simulink model "MMAE_leftlaneChange_behavior_identification"  (R2018b)
settings: Solver=FixedStepAuto  StartTime=0.0  StopTime=15  FixedStep=1e-3  RelTol=1e-3
values from neighbouring files (symbols this model uses):
  P_init = 1    [initialization.m]
  Ts_bp = 0.1    [initialization.m]    (also in laneChangeSinusoidalFcn.m = 0.01; laneChangeSinusoidalJacobianFcn.m = 0.01; leftLaneChangeParametricFcn.m = 0.01; leftLaneChangeParametricWithAccFcn.m = 0.01)
  vx = X(2)    [cv_model_fun.m]    (also in initialization.m = 10)
  vy = X(4)    [cv_model_fun.m]    (also in initialization.m = 0)
  x = X(1)    [KinematicBicycleModel.m]    (also in SimplifiedKinematicBicycleModel.m; behavior_model.m = 0:0.01:20; cca_model_fun.m; ctra_model_fun.m)
  y = X(2)    [KinematicBicycleModel.m]    (also in SimplifiedKinematicBicycleModel.m; behavior_model.m = [distances velocities]; cca_model_fun.m; ctra_model_fun.m)
libraries: simulink x5
settings Model: Creator=jasprit  LastModifiedBy=jasprit
settings SFSimCC: SimUseLocalCustomCode=off
settings RTWCC: RTWUseLocalCustomCode=off

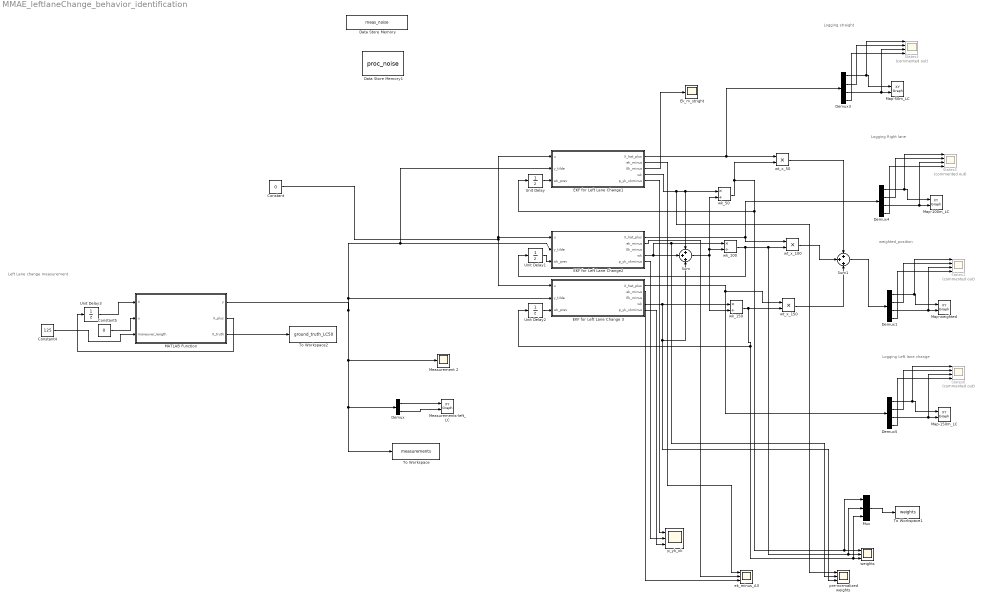
== system MMAE_leftlaneChange_behavior_identification ==
  note: Logging Left lane change
  note: Logging straight
  note: Logging Right lane
  note: weighted_position
  note: Left Lane change measurement
  Constant : Constant  Value=0
  Constant4 : Constant  Value=125  SampleTime=-1
  Constant5 : Constant  Value=0  SampleTime=-1
  Data Store Memory : DataStoreMemory  DataStoreName=meas_noise  ReadBeforeWriteMsg=warning  WriteAfterWriteMsg=warning  WriteAfterReadMsg=warning  InitialValue=[0.0025 0.0025]  ShowAdditionalParam=off  OutDataTypeStr=double
  Data Store Memory1 : DataStoreMemory  DataStoreName=proc_noise  ReadBeforeWriteMsg=warning  WriteAfterWriteMsg=warning  WriteAfterReadMsg=warning  InitialValue=[0.01 0.01 0.01 0.01]  ShowAdditionalParam=off  OutDataTypeStr=double
  Demux : Demux  Outputs=2
  Demux{1,3..5} (4 alike) : Demux
  EKF for Left Lane Change 3 : Subsystem
  EKF for Left Lane Change1 : Subsystem
  EKF for Left Lane Change2 : Subsystem
  Ek_m_stright : Scope
  MATLAB Function : MATLAB Function  TreatAsAtomicUnit=on
  Map-100m_LC : simulink/Sinks/XY Graph  xmin=-1  xmax=200  ymin=-5  ymax=5  st=-1
  Map-150m_LC : simulink/Sinks/XY Graph  xmin=-1  xmax=200  ymin=-5  ymax=5  st=-1
  Map-50m_LC : simulink/Sinks/XY Graph  xmin=-1  xmax=200  ymin=-5  ymax=5  st=-1
  Map-weighted : simulink/Sinks/XY Graph  xmin=-1  xmax=200  ymin=-5  ymax=5  st=-1
  Measurement 2 : Scope
  Measurements-left_LC : simulink/Sinks/XY Graph  xmin=-1  xmax=200  ymin=-5  ymax=5  st=-1
  Mux : Mux  Inputs=3
  States{1,4..6} (4 alike) : Scope  Commented=on  NumInputPorts=4
  Sum : Sum  Inputs=+++
  Sum1 : Sum  Inputs=+++
  To Workspace : ToWorkspace  VariableName=measurements  SaveFormat=Timeseries  SampleTime=Ts_bp
  To Workspace1 : ToWorkspace  VariableName=weights  SaveFormat=Timeseries  SampleTime=Ts_bp
  To Workspace2 : ToWorkspace  VariableName=ground_truth_LC50  SaveFormat=Timeseries  SampleTime=Ts_bp
  Unit Delay : UnitDelay  InitialCondition=1/3  SampleTime=-1
  Unit Delay1 : UnitDelay  InitialCondition=1/3  SampleTime=-1
  Unit Delay2 : UnitDelay  InitialCondition=1/3  SampleTime=-1
  Unit Delay3 : UnitDelay  InitialCondition=[x vx y vy]  SampleTime=Ts_bp
  ek_minus_All : Scope  NumInputPorts=3
  p_yk_xk : Scope  NumInputPorts=3
  pre-normalized weights : Scope  NumInputPorts=3
  weights : Scope  NumInputPorts=3
  wk_100 : Product  Inputs=*/
  wk_150 : Product  Inputs=*/
  wk_50 : Product  Inputs=*/
  wt_x_100 : Product  Inputs=**
  wt_x_150 : Product  Inputs=**
  wt_x_50 : Product  Inputs=**
  wires:
  Demux3/1 -> States4/1, Map-50m_LC/1
  Demux3/4 -> States4/4
  Demux3/2 -> States4/2
  Demux3/3 -> Map-50m_LC/2, States4/3
  Constant/1 -> EKF for Left Lane Change2/1(u), EKF for Left Lane Change1/1(u), EKF for Left Lane Change 3/1(u)
  Demux4/1 -> States5/1, Map-100m_LC/1
  Demux4/2 -> States5/2
  Demux4/4 -> States5/4
  Demux4/3 -> Map-100m_LC/2, States5/3
  Demux5/1 -> States6/1, Map-150m_LC/1
  Demux5/4 -> States6/4
  Demux5/3 -> Map-150m_LC/2, States6/3
  Demux5/2 -> States6/2
  EKF for Left Lane Change 3/1(X_hat_plus) -> wt_x_150/1, Demux5/1
  EKF for Left Lane Change2/1(X_hat_plus) -> Demux4/1, wt_x_100/1
  EKF for Left Lane Change 3/4(wk) -> wk_150/1, pre-normalized weights/3, Sum/3
  EKF for Left Lane Change2/4(wk) -> pre-normalized weights/2, wk_100/1, Sum/2
  Sum/1 -> wk_150/2, wk_50/2, wk_100/2
  wk_50/1 -> Unit Delay/1, Mux/1, weights/1, wt_x_50/2
  wk_100/1 -> Unit Delay1/1, Mux/2, weights/2, wt_x_100/2
  wt_x_100/1 -> Sum1/2
  wt_x_50/1 -> Sum1/1
  wt_x_150/1 -> Sum1/3
  Demux1/1 -> States1/1, Map-weighted/1
  Demux1/4 -> States1/4
  Demux1/2 -> States1/2
  Demux1/3 -> States1/3, Map-weighted/2
  Sum1/1 -> Demux1/1
  Unit Delay/1 -> EKF for Left Lane Change1/3(wk_prev)
  Unit Delay1/1 -> EKF for Left Lane Change2/3(wk_prev)
  Unit Delay2/1 -> EKF for Left Lane Change 3/3(wk_prev)
  EKF for Left Lane Change2/2(ek_minus) -> ek_minus_All/2
  EKF for Left Lane Change 3/2(ek_minus) -> ek_minus_All/3
  MATLAB Function/1(y) -> Measurement 2/1, Demux/1, To Workspace/1, EKF for Left Lane Change 3/2(y_tilde), EKF for Left Lane Change1/2(y_tilde), EKF for Left Lane Change2/2(y_tilde)
  EKF for Left Lane Change2/5(p_yk_xkminus) -> p_yk_xk/2
  EKF for Left Lane Change 3/5(p_yk_xkminus) -> p_yk_xk/3
  EKF for Left Lane Change1/1(X_hat_plus) -> Demux3/1, wt_x_50/1
  EKF for Left Lane Change1/2(ek_minus) -> ek_minus_All/1
  EKF for Left Lane Change1/4(wk) -> pre-normalized weights/1, wk_50/1, Sum/1
  EKF for Left Lane Change1/5(p_yk_xkminus) -> p_yk_xk/1
  EKF for Left Lane Change1/3(Ek_minus) -> Ek_m_stright/1
  wk_150/1 -> Unit Delay2/1, Mux/3, weights/3, wt_x_150/2
  Mux/1 -> To Workspace1/1
  Constant5/1 -> MATLAB Function/2(u)
  MATLAB Function/2(X_plus) -> Unit Delay3/1
  Unit Delay3/1 -> MATLAB Function/1(X)
  Constant4/1 -> MATLAB Function/3(maneuver_length)
  Demux/1 -> Measurements-left_LC/1
  Demux/2 -> Measurements-left_LC/2
  MATLAB Function/3(X_truth) -> To Workspace2/1

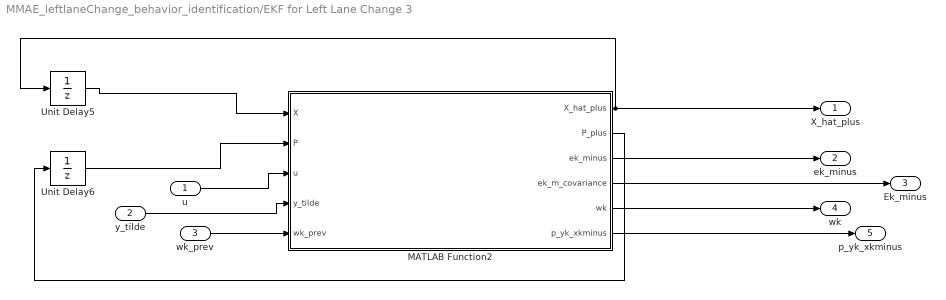
== system MMAE_leftlaneChange_behavior_identification/EKF for Left Lane Change 3 ==
  u : Inport
  y_tilde : Inport  Port=2
  wk_prev : Inport  Port=3
  MATLAB Function2 : MATLAB Function  TreatAsAtomicUnit=on
  Unit Delay5 : UnitDelay  InitialCondition=[x vx y vy]  SampleTime=-1
  Unit Delay6 : UnitDelay  InitialCondition=P_init  SampleTime=-1
  X_hat_plus : Outport
  ek_minus : Outport  Port=2
  Ek_minus : Outport  Port=3
  wk : Outport  Port=4
  p_yk_xkminus : Outport  Port=5
  wires:
  MATLAB Function2/2(P_plus) -> Unit Delay6/1
  u/1 -> MATLAB Function2/3(u)
  y_tilde/1 -> MATLAB Function2/4(y_tilde)
  MATLAB Function2/1(X_hat_plus) -> X_hat_plus/1, Unit Delay5/1
  Unit Delay5/1 -> MATLAB Function2/1(X)
  Unit Delay6/1 -> MATLAB Function2/2(P)
  MATLAB Function2/3(ek_minus) -> ek_minus/1
  MATLAB Function2/4(ek_m_covariance) -> Ek_minus/1
  MATLAB Function2/5(wk) -> wk/1
  MATLAB Function2/6(p_yk_xkminus) -> p_yk_xkminus/1
  wk_prev/1 -> MATLAB Function2/5(wk_prev)

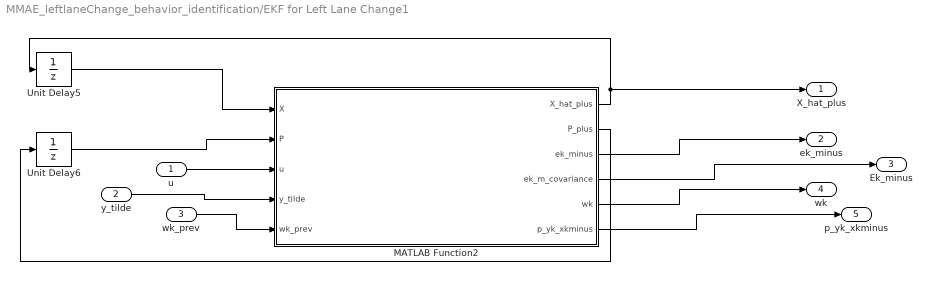
== system MMAE_leftlaneChange_behavior_identification/EKF for Left Lane Change1 ==
  u : Inport
  y_tilde : Inport  Port=2
  wk_prev : Inport  Port=3
  MATLAB Function2 : MATLAB Function  TreatAsAtomicUnit=on
  Unit Delay5 : UnitDelay  InitialCondition=[x vx y vy]  SampleTime=-1
  Unit Delay6 : UnitDelay  InitialCondition=P_init  SampleTime=-1
  X_hat_plus : Outport
  ek_minus : Outport  Port=2
  Ek_minus : Outport  Port=3
  wk : Outport  Port=4
  p_yk_xkminus : Outport  Port=5
  wires:
  MATLAB Function2/2(P_plus) -> Unit Delay6/1
  u/1 -> MATLAB Function2/3(u)
  y_tilde/1 -> MATLAB Function2/4(y_tilde)
  MATLAB Function2/1(X_hat_plus) -> Unit Delay5/1, X_hat_plus/1
  Unit Delay5/1 -> MATLAB Function2/1(X)
  Unit Delay6/1 -> MATLAB Function2/2(P)
  MATLAB Function2/3(ek_minus) -> ek_minus/1
  MATLAB Function2/4(ek_m_covariance) -> Ek_minus/1
  MATLAB Function2/5(wk) -> wk/1
  MATLAB Function2/6(p_yk_xkminus) -> p_yk_xkminus/1
  wk_prev/1 -> MATLAB Function2/5(wk_prev)

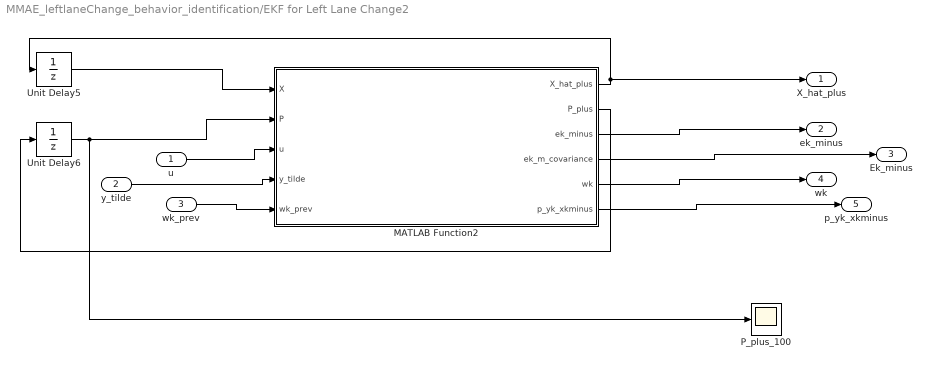
== system MMAE_leftlaneChange_behavior_identification/EKF for Left Lane Change2 ==
  u : Inport
  y_tilde : Inport  Port=2
  wk_prev : Inport  Port=3
  MATLAB Function2 : MATLAB Function  TreatAsAtomicUnit=on
  P_plus_100 : Scope
  Unit Delay5 : UnitDelay  InitialCondition=[x vx y vy]  SampleTime=-1
  Unit Delay6 : UnitDelay  InitialCondition=P_init  SampleTime=-1
  X_hat_plus : Outport
  ek_minus : Outport  Port=2
  Ek_minus : Outport  Port=3
  wk : Outport  Port=4
  p_yk_xkminus : Outport  Port=5
  wires:
  MATLAB Function2/2(P_plus) -> Unit Delay6/1
  u/1 -> MATLAB Function2/3(u)
  y_tilde/1 -> MATLAB Function2/4(y_tilde)
  MATLAB Function2/1(X_hat_plus) -> Unit Delay5/1, X_hat_plus/1
  Unit Delay5/1 -> MATLAB Function2/1(X)
  Unit Delay6/1 -> P_plus_100/1, MATLAB Function2/2(P)
  MATLAB Function2/3(ek_minus) -> ek_minus/1
  MATLAB Function2/4(ek_m_covariance) -> Ek_minus/1
  MATLAB Function2/5(wk) -> wk/1
  MATLAB Function2/6(p_yk_xkminus) -> p_yk_xkminus/1
  wk_prev/1 -> MATLAB Function2/5(wk_prev)

== matlab function MMAE_leftlaneChange_behavior_identification/EKF for Left Lane Change2/MATLAB Function2 ==
  data: X input; P input; u input; X_hat_plus output; y_tilde input; P_plus output; ek_minus output; ek_m_covariance output; wk output; p_yk_xkminus output; wk_prev input; meas_noise data_store_memory; proc_noise data_store_memory
function [X_hat_plus, P_plus, ek_minus, ek_m_covariance, wk, p_yk_xkminus] = EKFLeftLaneChangeCustom(X, P, u, y_tilde, wk_prev)

    maneuver_length = 100;  %meters
    lane_center_to_center_distance = 3.5;   %meters
    
    %%
    %TODO: See how can this be moved out of the function later
    %sampling time
    Ts = 0.01;

    % measurement noise covariance
%     R = [0.2 0; 0 0.2];
%     R = [0.0025 0; 0 0.0025];
    global meas_noise;
    R = diag(meas_noise);
    
    % process noise covariance
%     Q = diag([0.5 5.0 0.5 5.0]);
%     Q = diag([0.001 0.001 0.001 0.001]);
    global proc_noise;
    Q = diag(proc_noise);

    % states - X = [x vx y vy] -     
    Ck = [1 0 0 0; 0 0 1 0];

    F = leftLaneChangeParametricJacobianFcn(X, u, maneuver_length, lane_center_to_center_distance);
    %%
    % Now estimate states using kalman filter
    
    %predict
    xhat_minus = leftLaneChangeParametricFcn(X, u, maneuver_length, lane_center_to_center_distance);
    P_minus = (F * P * F') + Ts*Q;
    yhat_minus = Ck * xhat_minus;

    %correct
    ek_minus = y_tilde - yhat_minus;    %residual
    ek_m_covariance = Ck * P_minus *Ck' + R;    %residual covariance
    K = P_minus * Ck' * inv(ek_m_covariance);
    X_hat_plus = xhat_minus + K * ek_minus;
    P_plus = (eye(4) - K * Ck) * P_minus;
    
    %calculate MMAE weights
    p_yk_xkminus = 1/sqrt(det(2*pi*ek_m_covariance))*exp(-1/2 * ek_minus'* inv(ek_m_covariance) * ek_minus);
    wk = wk_prev * p_yk_xkminus;

    
end

== matlab function MMAE_leftlaneChange_behavior_identification/EKF for Left Lane Change1/MATLAB Function2 ==
  data: X input; P input; u input; X_hat_plus output; y_tilde input; P_plus output; ek_minus output; ek_m_covariance output; wk output; p_yk_xkminus output; wk_prev input; meas_noise data_store_memory; proc_noise data_store_memory
function [X_hat_plus, P_plus, ek_minus, ek_m_covariance, wk, p_yk_xkminus] = EKFLeftLaneChangeCustom(X, P, u, y_tilde, wk_prev)

    maneuver_length = 50;  %meters
    lane_center_to_center_distance = 3.5;   %meters
    
    %%
    %TODO: See how can this be moved out of the function later
    %sampling time
    Ts = 0.01;

    % measurement noise covariance
%     R = [0.2 0; 0 0.2];
%    R = [0.0025 0; 0 0.0025];
    global meas_noise;
     R = diag(meas_noise);
   
    % process noise covariance
%     Q = diag([0.5 5.0 0.5 5.0]);
%     Q = diag([0.001 0.001 0.001 0.001]);
    global proc_noise;
    Q = diag(proc_noise);
    
    % states - X = [x vx y vy] -     
    Ck = [1 0 0 0; 0 0 1 0];

    F = leftLaneChangeParametricJacobianFcn(X, u, maneuver_length, lane_center_to_center_distance);
    %%
    % Now estimate states using kalman filter
    
    %predict
    xhat_minus = leftLaneChangeParametricFcn(X, u, maneuver_length, lane_center_to_center_distance);
    P_minus = (F * P * F') + Ts*Q;
    yhat_minus = Ck * xhat_minus;

    %correct
    ek_minus = y_tilde - yhat_minus;    %residual
    ek_m_covariance = Ck * P_minus *Ck' + R;    %residual covariance
    K = P_minus * Ck' * inv(ek_m_covariance);
    X_hat_plus = xhat_minus + K * ek_minus;
    P_plus = (eye(4) - K * Ck) * P_minus;
    
    %calculate MMAE weights
    p_yk_xkminus = 1/sqrt(det(2*pi*ek_m_covariance))*exp(-1/2 * ek_minus'* inv(ek_m_covariance) * ek_minus);
    wk = wk_prev * p_yk_xkminus;

    
end

== matlab function MMAE_leftlaneChange_behavior_identification/EKF for Left Lane Change 3/MATLAB Function2 ==
  data: X input; P input; u input; X_hat_plus output; y_tilde input; P_plus output; ek_minus output; ek_m_covariance output; wk output; p_yk_xkminus output; wk_prev input; meas_noise data_store_memory; proc_noise data_store_memory
function [X_hat_plus, P_plus, ek_minus, ek_m_covariance, wk, p_yk_xkminus] = EKFLeftLaneChangeCustom(X, P, u, y_tilde, wk_prev)

    maneuver_length = 150;  %meters
    lane_center_to_center_distance = 3.5;   %meters
    
    %%
    %TODO: See how can this be moved out of the function later
    %sampling time
    Ts = 0.01;

    % measurement noise covariance
%     R = [0.2 0; 0 0.2];
%     R = [0.0025 0; 0 0.0025];
    global meas_noise;
    R = diag(meas_noise);
    
    % process noise covariance
%     Q = diag([0.5 5.0 0.5 5.0]);
%     Q = diag([0.001 0.001 0.001 0.001]);
    global proc_noise;
    Q = diag(proc_noise);

    % states - X = [x vx y vy] -     
    Ck = [1 0 0 0; 0 0 1 0];

    F = leftLaneChangeParametricJacobianFcn(X, u, maneuver_length, lane_center_to_center_distance);
    %%
    % Now estimate states using kalman filter
    
    %predict
    xhat_minus = leftLaneChangeParametricFcn(X, u, maneuver_length, lane_center_to_center_distance);
    P_minus = (F * P * F') + Ts*Q;
    yhat_minus = Ck * xhat_minus;

    %correct
    ek_minus = y_tilde - yhat_minus;    %residual
    ek_m_covariance = Ck * P_minus *Ck' + R;    %residual covariance
    K = P_minus * Ck' * inv(ek_m_covariance);
    X_hat_plus = xhat_minus + K * ek_minus;
    P_plus = (eye(4) - K * Ck) * P_minus;
    
    %calculate MMAE weights
    p_yk_xkminus = 1/sqrt(det(2*pi*ek_m_covariance))*exp(-1/2 * ek_minus'* inv(ek_m_covariance) * ek_minus);
    wk = wk_prev * p_yk_xkminus;

    
end

== matlab function MMAE_leftlaneChange_behavior_identification/MATLAB Function ==
  data: X input; u input; y output; X_plus output; maneuver_length input; meas_noise data_store_memory; proc_noise data_store_memory; X_truth output
function [y, X_plus, X_truth]= measurementsForLaneChange(X, u, maneuver_length)

    Ts_bp = 0.01;
%     maneuver_length = 150;  %m
    lane_center_to_center_distance = 3.5;   %meters

    % states - X = [x vx y vy] -     
    Ck = [1 0 0 0; 0 0 1 0];

    % measurement noise std_dev
%      R_sigma = [0 0; 0 0];
%    R_sigma = [0.05 0; 0 0.05];
    global meas_noise;
    R_sigma = diag(sqrt(meas_noise));
    
    % process noise std dev
   sigma_matrix = diag([0 0 0 0]);
%     sigma_matrix = diag([0.032 0.032 0.032 0.032]);
%     global proc_noise;
%     sigma_matrix = diag(sqrt(proc_noise));

%     if t < 15
%         Ak = [1 Ts 0 0; 0 1 0 0; 0 0 1 Ts; 0 0 0 1];
%         Bk = 0;
%         X_plus = Ak * X + Bk * u + sqrt(Ts) * sigma_matrix * randn(4,1);
%     else
        X_truth = leftLaneChangeParametricFcn(X, u, maneuver_length, lane_center_to_center_distance);
        X_plus = X_truth + sqrt(Ts_bp)*sigma_matrix*randn(4,1);    
%     end
    
    y = Ck * X_plus + R_sigma * randn(2,1);
    
end
